simulink model "Digital-Memory-Architecture"  (R2024b)
settings: Solver=VariableStepAuto  StartTime=0.0  StopTime=10.0  RelTol=1e-3
libraries: simulink_extras x129
(part 1 of 5)
settings Model: Creator=suhanoner  LastModifiedBy=suhanoner

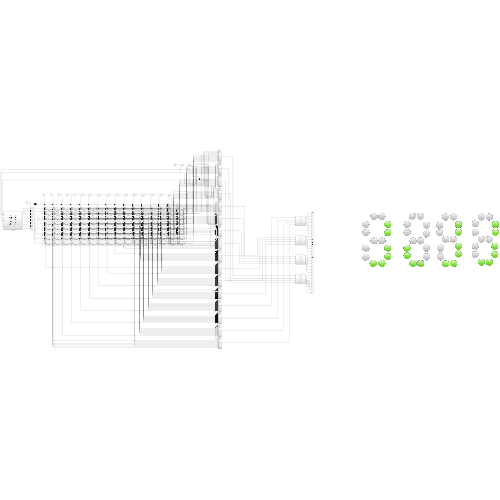
[thumbnail: Simulink's stored preview of the top-level diagram]
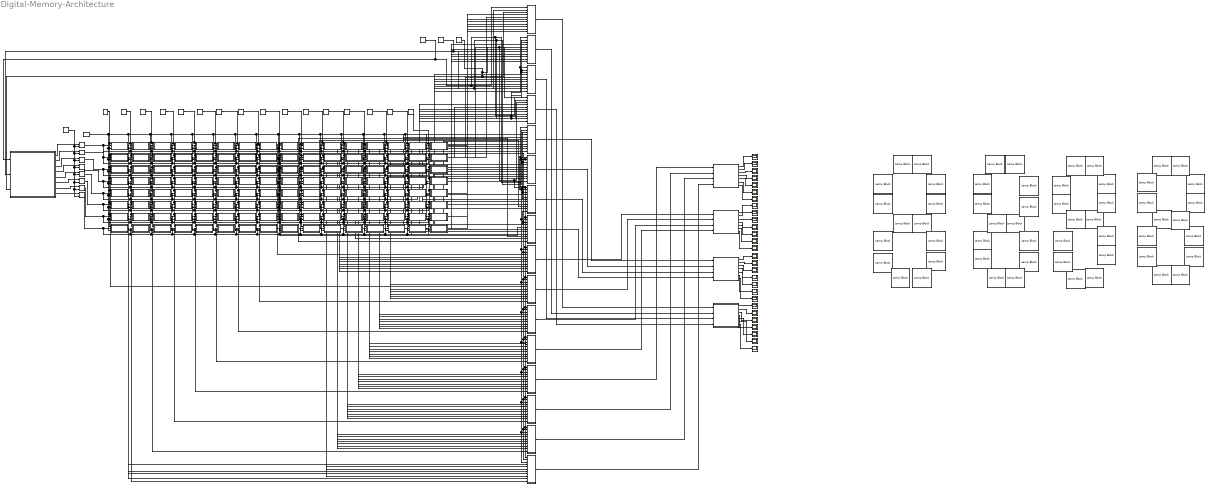
== system Digital-Memory-Architecture ==
  3 to 8 Decoder : Subsystem
  8to1MUX : Subsystem
  8to1MUX1 : Subsystem
  8to1MUX10 : Subsystem
  8to1MUX11 : Subsystem
  8to1MUX12 : Subsystem
  8to1MUX13 : Subsystem
  8to1MUX14 : Subsystem
  8to1MUX15 : Subsystem
  8to1MUX2 : Subsystem
  8to1MUX3 : Subsystem
  8to1MUX4 : Subsystem
  8to1MUX5 : Subsystem
  8to1MUX6 : Subsystem
  8to1MUX7 : Subsystem
  8to1MUX8 : Subsystem
  8to1MUX9 : Subsystem
  Adress0 : Constant
  Adress1 : Constant  Value=0
  Adress2 : Constant  Value=0
  BitCell1 : Subsystem
  BitCell10 : Subsystem
  BitCell100 : Subsystem
  BitCell101 : Subsystem
  BitCell102 : Subsystem
  BitCell103 : Subsystem
  BitCell104 : Subsystem
  BitCell105 : Subsystem
  BitCell106 : Subsystem
  BitCell107 : Subsystem
  BitCell108 : Subsystem
  BitCell109 : Subsystem
  BitCell11 : Subsystem
  BitCell110 : Subsystem
  BitCell111 : Subsystem
  BitCell112 : Subsystem
  BitCell113 : Subsystem
  BitCell114 : Subsystem
  BitCell115 : Subsystem
  BitCell116 : Subsystem
  BitCell117 : Subsystem
  BitCell118 : Subsystem
  BitCell119 : Subsystem
  BitCell12 : Subsystem
  BitCell120 : Subsystem
  BitCell121 : Subsystem
  BitCell122 : Subsystem
  BitCell123 : Subsystem
  BitCell124 : Subsystem
  BitCell125 : Subsystem
  BitCell126 : Subsystem
  BitCell127 : Subsystem
  BitCell128 : Subsystem
  BitCell13 : Subsystem
  BitCell14 : Subsystem
  BitCell15 : Subsystem
  BitCell16 : Subsystem
  BitCell17 : Subsystem
  BitCell18 : Subsystem
  BitCell19 : Subsystem
  BitCell2 : Subsystem
  BitCell20 : Subsystem
  BitCell21 : Subsystem
  BitCell22 : Subsystem
  BitCell23 : Subsystem
  BitCell24 : Subsystem
  BitCell25 : Subsystem
  BitCell26 : Subsystem
  BitCell27 : Subsystem
  BitCell28 : Subsystem
  BitCell29 : Subsystem
  BitCell3 : Subsystem
  BitCell30 : Subsystem
  BitCell31 : Subsystem
  BitCell32 : Subsystem
  BitCell33 : Subsystem
  BitCell34 : Subsystem
  BitCell35 : Subsystem
  BitCell36 : Subsystem
  BitCell37 : Subsystem
  BitCell38 : Subsystem
  BitCell39 : Subsystem
  BitCell4 : Subsystem
  BitCell40 : Subsystem
  BitCell41 : Subsystem
  BitCell42 : Subsystem
  BitCell43 : Subsystem
  BitCell44 : Subsystem
  BitCell45 : Subsystem
  BitCell46 : Subsystem
  BitCell47 : Subsystem
  BitCell48 : Subsystem
  BitCell49 : Subsystem
  BitCell5 : Subsystem
  BitCell50 : Subsystem
  BitCell51 : Subsystem
  BitCell52 : Subsystem
  BitCell53 : Subsystem
  BitCell54 : Subsystem
  BitCell55 : Subsystem
  BitCell56 : Subsystem
  BitCell57 : Subsystem
  BitCell58 : Subsystem
  BitCell59 : Subsystem
  BitCell6 : Subsystem
  BitCell60 : Subsystem
  BitCell61 : Subsystem
  BitCell62 : Subsystem
  BitCell63 : Subsystem
  BitCell64 : Subsystem
  BitCell65 : Subsystem
  BitCell66 : Subsystem
  BitCell67 : Subsystem
  BitCell68 : Subsystem
  BitCell69 : Subsystem
  BitCell7 : Subsystem
  BitCell70 : Subsystem
  BitCell71 : Subsystem
  BitCell72 : Subsystem
  BitCell73 : Subsystem
  BitCell74 : Subsystem
  BitCell75 : Subsystem
  BitCell76 : Subsystem
  BitCell77 : Subsystem
  BitCell78 : Subsystem
  BitCell79 : Subsystem
  BitCell8 : Subsystem
  BitCell80 : Subsystem
  BitCell81 : Subsystem
  BitCell82 : Subsystem
  BitCell83 : Subsystem
  BitCell84 : Subsystem
  BitCell85 : Subsystem
  BitCell86 : Subsystem
  BitCell87 : Subsystem
  BitCell88 : Subsystem
  BitCell89 : Subsystem
  BitCell9 : Subsystem
  BitCell90 : Subsystem
  BitCell91 : Subsystem
  BitCell92 : Subsystem
  BitCell93 : Subsystem
  BitCell94 : Subsystem
  BitCell95 : Subsystem
  BitCell96 : Subsystem
  BitCell97 : Subsystem
  BitCell98 : Subsystem
  BitCell99 : Subsystem
  Clock : simulink_extras/Flip Flops/Clock  period=2
  D_in{,1..4,7..15} (14 alike) : Constant
  D_in5 : Constant  Value=0
  D_in6 : Constant  Value=0
  Lamp{,1..55} (56 alike) : LampBlock  LabelPosition=Hide
  Logical Operator{,1..7} (8 alike) : Logic  AllPortsSameDT=off  OutDataTypeStr=boolean
  R/W : Constant
  Scope{,1..27} (28 alike) : Scope
  Subsystem2 : Subsystem
  Subsystem3 : Subsystem
  Subsystem4 : Subsystem
  Subsystem5 : Subsystem
  wires:
  3 to 8 Decoder/1(Y0) -> Logical Operator/1
  3 to 8 Decoder/2(Y1) -> Logical Operator1/1
  3 to 8 Decoder/3(Y2) -> Logical Operator2/1
  3 to 8 Decoder/4(Y3) -> Logical Operator3/1
  3 to 8 Decoder/5(Y4) -> Logical Operator4/1
  3 to 8 Decoder/6(Y5) -> Logical Operator5/1
  3 to 8 Decoder/7(Y6) -> Logical Operator6/1
  3 to 8 Decoder/8(Y7) -> Logical Operator7/1
  R/W/1 -> Logical Operator7/2, Logical Operator6/2, Logical Operator5/2, Logical Operator4/2, Logical Operator3/2, Logical Operator2/2, Logical Operator1/2, Logical Operator/2
  D_in/1 -> BitCell1/1(D), BitCell9/1(D), BitCell17/1(D), BitCell25/1(D), BitCell33/1(D), BitCell41/1(D), BitCell57/1(D), BitCell49/1(D)
  D_in1/1 -> BitCell2/1(D), BitCell10/1(D), BitCell18/1(D), BitCell26/1(D), BitCell34/1(D), BitCell42/1(D), BitCell58/1(D), BitCell50/1(D)
  D_in2/1 -> BitCell3/1(D), BitCell11/1(D), BitCell19/1(D), BitCell27/1(D), BitCell35/1(D), BitCell43/1(D), BitCell59/1(D), BitCell51/1(D)
  D_in8/1 -> BitCell64/1(D), BitCell100/1(D), BitCell15/1(D), BitCell24/1(D), BitCell39/1(D), BitCell48/1(D), BitCell128/1(D), BitCell91/1(D)
  D_in10/1 -> BitCell102/1(D), BitCell67/1(D), BitCell75/1(D), BitCell83/1(D), BitCell87/1(D), BitCell98/1(D), BitCell110/1(D), BitCell119/1(D)
  Logical Operator/1 -> BitCell1/2(WE), BitCell2/2(WE), BitCell3/2(WE), BitCell4/2(WE), BitCell5/2(WE), BitCell46/2(WE), BitCell55/2(WE), BitCell65/2(WE), BitCell64/2(WE), BitCell93/2(WE), BitCell102/2(WE), BitCell101/2(WE), BitCell99/2(WE), BitCell125/2(WE), BitCell71/2(WE), BitCell70/2(WE)
  Logical Operator4/1 -> BitCell33/2(WE), BitCell34/2(WE), BitCell35/2(WE), BitCell36/2(WE), BitCell37/2(WE), BitCell30/2(WE), BitCell40/2(WE), BitCell47/2(WE), BitCell39/2(WE), BitCell85/2(WE), BitCell87/2(WE), BitCell84/2(WE), BitCell96/2(WE), BitCell120/2(WE), BitCell122/2(WE), BitCell116/2(WE)
  Logical Operator2/1 -> BitCell17/2(WE), BitCell18/2(WE), BitCell19/2(WE), BitCell20/2(WE), BitCell21/2(WE), BitCell14/2(WE), BitCell16/2(WE), BitCell23/2(WE), BitCell15/2(WE), BitCell74/2(WE), BitCell75/2(WE), BitCell68/2(WE), BitCell90/2(WE), BitCell107/2(WE), BitCell109/2(WE), BitCell106/2(WE)
  Logical Operator6/1 -> BitCell49/2(WE), BitCell50/2(WE), BitCell51/2(WE), BitCell52/2(WE), BitCell53/2(WE), BitCell54/2(WE), BitCell73/2(WE), BitCell82/2(WE), BitCell91/2(WE), BitCell103/2(WE), BitCell110/2(WE), BitCell111/2(WE), BitCell123/2(WE), BitCell72/2(WE), BitCell79/2(WE), BitCell78/2(WE)
  Logical Operator7/1 -> BitCell57/2(WE), BitCell58/2(WE), BitCell59/2(WE), BitCell60/2(WE), BitCell61/2(WE), BitCell62/2(WE), BitCell108/2(WE), BitCell117/2(WE), BitCell128/2(WE), BitCell118/2(WE), BitCell119/2(WE), BitCell121/2(WE), BitCell89/2(WE), BitCell81/2(WE), BitCell86/2(WE), BitCell88/2(WE)
  Clock/1 -> BitCell70/3(CLK), BitCell80/3(CLK), BitCell106/3(CLK), BitCell113/3(CLK), BitCell116/3(CLK), BitCell124/3(CLK), BitCell79/3(CLK), BitCell88/3(CLK), BitCell71/3(CLK), BitCell105/3(CLK), BitCell109/3(CLK), BitCell115/3(CLK), BitCell122/3(CLK), BitCell127/3(CLK), BitCell78/3(CLK), BitCell86/3(CLK), BitCell125/3(CLK), BitCell104/3(CLK), BitCell107/3(CLK), BitCell114/3(CLK), BitCell120/3(CLK), BitCell126/3(CLK), BitCell72/3(CLK), BitCell81/3(CLK), BitCell99/3(CLK), BitCell69/3(CLK), BitCell90/3(CLK), BitCell95/3(CLK), BitCell96/3(CLK), BitCell97/3(CLK), BitCell123/3(CLK), BitCell89/3(CLK), BitCell101/3(CLK), BitCell112/3(CLK), BitCell68/3(CLK), BitCell76/3(CLK), BitCell84/3(CLK), BitCell92/3(CLK), BitCell111/3(CLK), BitCell121/3(CLK), BitCell102/3(CLK), BitCell67/3(CLK), BitCell75/3(CLK), BitCell83/3(CLK), BitCell87/3(CLK), BitCell98/3(CLK), BitCell110/3(CLK), BitCell119/3(CLK), BitCell93/3(CLK), BitCell66/3(CLK), BitCell74/3(CLK), BitCell77/3(CLK), BitCell85/3(CLK), BitCell94/3(CLK), BitCell103/3(CLK), BitCell118/3(CLK), BitCell64/3(CLK), BitCell100/3(CLK), BitCell15/3(CLK), BitCell24/3(CLK), BitCell39/3(CLK), BitCell48/3(CLK), BitCell128/3(CLK), BitCell91/3(CLK), BitCell65/3(CLK), BitCell8/3(CLK), BitCell23/3(CLK), BitCell32/3(CLK), BitCell47/3(CLK), BitCell63/3(CLK), BitCell117/3(CLK), BitCell82/3(CLK), BitCell55/3(CLK), BitCell7/3(CLK), BitCell16/3(CLK), BitCell31/3(CLK), BitCell40/3(CLK), BitCell56/3(CLK), BitCell108/3(CLK), BitCell73/3(CLK), BitCell46/3(CLK), BitCell6/3(CLK), BitCell14/3(CLK), BitCell22/3(CLK), BitCell30/3(CLK), BitCell38/3(CLK), BitCell62/3(CLK), BitCell54/3(CLK), BitCell5/3(CLK), BitCell13/3(CLK), BitCell21/3(CLK), BitCell29/3(CLK), BitCell37/3(CLK), BitCell45/3(CLK), BitCell61/3(CLK), BitCell53/3(CLK), BitCell4/3(CLK), BitCell12/3(CLK), BitCell20/3(CLK), BitCell28/3(CLK), BitCell36/3(CLK), BitCell44/3(CLK), BitCell60/3(CLK), BitCell52/3(CLK), BitCell3/3(CLK), BitCell11/3(CLK), BitCell19/3(CLK), BitCell27/3(CLK), BitCell35/3(CLK), BitCell43/3(CLK), BitCell59/3(CLK), BitCell51/3(CLK), BitCell2/3(CLK), BitCell10/3(CLK), BitCell18/3(CLK), BitCell26/3(CLK), BitCell34/3(CLK), BitCell42/3(CLK), BitCell58/3(CLK), BitCell50/3(CLK), BitCell1/3(CLK), BitCell9/3(CLK), BitCell17/3(CLK), BitCell25/3(CLK), BitCell33/3(CLK), BitCell41/3(CLK), BitCell57/3(CLK), BitCell49/3(CLK)
  Logical Operator1/1 -> BitCell9/2(WE), BitCell10/2(WE), BitCell11/2(WE), BitCell12/2(WE), BitCell13/2(WE), BitCell6/2(WE), BitCell7/2(WE), BitCell8/2(WE), BitCell100/2(WE), BitCell66/2(WE), BitCell67/2(WE), BitCell112/2(WE), BitCell69/2(WE), BitCell104/2(WE), BitCell80/2(WE), BitCell105/2(WE)
  Logical Operator3/1 -> BitCell25/2(WE), BitCell26/2(WE), BitCell27/2(WE), BitCell28/2(WE), BitCell29/2(WE), BitCell22/2(WE), BitCell31/2(WE), BitCell32/2(WE), BitCell24/2(WE), BitCell77/2(WE), BitCell83/2(WE), BitCell76/2(WE), BitCell95/2(WE), BitCell114/2(WE), BitCell115/2(WE), BitCell113/2(WE)
  Logical Operator5/1 -> BitCell41/2(WE), BitCell42/2(WE), BitCell43/2(WE), BitCell44/2(WE), BitCell45/2(WE), BitCell38/2(WE), BitCell56/2(WE), BitCell63/2(WE), BitCell48/2(WE), BitCell94/2(WE), BitCell98/2(WE), BitCell92/2(WE), BitCell97/2(WE), BitCell126/2(WE), BitCell127/2(WE), BitCell124/2(WE)
  D_in9/1 -> BitCell93/1(D), BitCell66/1(D), BitCell74/1(D), BitCell77/1(D), BitCell85/1(D), BitCell94/1(D), BitCell103/1(D), BitCell118/1(D)
  D_in3/1 -> BitCell12/1(D), BitCell20/1(D), BitCell28/1(D), BitCell36/1(D), BitCell44/1(D), BitCell60/1(D), BitCell52/1(D), BitCell4/1(D)
  D_in4/1 -> BitCell5/1(D), BitCell13/1(D), BitCell21/1(D), BitCell29/1(D), BitCell37/1(D), BitCell45/1(D), BitCell61/1(D), BitCell53/1(D)
  D_in5/1 -> BitCell6/1(D), BitCell14/1(D), BitCell22/1(D), BitCell30/1(D), BitCell38/1(D), BitCell54/1(D), BitCell62/1(D), BitCell46/1(D)
  D_in6/1 -> BitCell7/1(D), BitCell16/1(D), BitCell31/1(D), BitCell40/1(D), BitCell56/1(D), BitCell108/1(D), BitCell73/1(D), BitCell55/1(D)
  D_in7/1 -> BitCell8/1(D), BitCell23/1(D), BitCell32/1(D), BitCell47/1(D), BitCell63/1(D), BitCell117/1(D), BitCell82/1(D), BitCell65/1(D)
  D_in13/1 -> BitCell125/1(D), BitCell104/1(D), BitCell107/1(D), BitCell114/1(D), BitCell120/1(D), BitCell126/1(D), BitCell72/1(D), BitCell81/1(D)
  D_in14/1 -> BitCell105/1(D), BitCell109/1(D), BitCell115/1(D), BitCell122/1(D), BitCell127/1(D), BitCell86/1(D), BitCell78/1(D), BitCell71/1(D)
  D_in12/1 -> BitCell69/1(D), BitCell90/1(D), BitCell95/1(D), BitCell96/1(D), BitCell97/1(D), BitCell123/1(D), BitCell89/1(D), BitCell99/1(D)
  D_in15/1 -> BitCell80/1(D), BitCell106/1(D), BitCell113/1(D), BitCell116/1(D), BitCell124/1(D), BitCell79/1(D), BitCell88/1(D), BitCell70/1(D)
  D_in11/1 -> BitCell101/1(D), BitCell112/1(D), BitCell68/1(D), BitCell76/1(D), BitCell84/1(D), BitCell92/1(D), BitCell111/1(D), BitCell121/1(D)
  BitCell70/1(Q) -> 8to1MUX/4(D0)
  BitCell80/1(Q) -> 8to1MUX/5(D1)
  BitCell106/1(Q) -> 8to1MUX/6(D2)
  BitCell113/1(Q) -> 8to1MUX/7(D3)
  BitCell116/1(Q) -> 8to1MUX/8(D4)
  BitCell124/1(Q) -> 8to1MUX/9(D5)
  BitCell79/1(Q) -> 8to1MUX/10(D6)
  BitCell88/1(Q) -> 8to1MUX/11(D7)
  BitCell127/1(Q) -> 8to1MUX1/9(D5)
  BitCell122/1(Q) -> 8to1MUX1/8(D4)
  BitCell109/1(Q) -> 8to1MUX1/6(D2)
  BitCell105/1(Q) -> 8to1MUX1/5(D1)
  BitCell115/1(Q) -> 8to1MUX1/7(D3)
  BitCell78/1(Q) -> 8to1MUX1/10(D6)
  BitCell86/1(Q) -> 8to1MUX1/11(D7)
  BitCell71/1(Q) -> 8to1MUX1/4(D0)
  BitCell120/1(Q) -> 8to1MUX2/8(D4)
  BitCell114/1(Q) -> 8to1MUX2/7(D3)
  BitCell107/1(Q) -> 8to1MUX2/6(D2)
  BitCell81/1(Q) -> 8to1MUX2/11(D7)
  BitCell125/1(Q) -> 8to1MUX2/4(D0)
  BitCell104/1(Q) -> 8to1MUX2/5(D1)
  BitCell72/1(Q) -> 8to1MUX2/10(D6)
  BitCell126/1(Q) -> 8to1MUX2/9(D5)
  BitCell96/1(Q) -> 8to1MUX3/8(D4)
  BitCell95/1(Q) -> 8to1MUX3/7(D3)
  BitCell90/1(Q) -> 8to1MUX3/6(D2)
  BitCell89/1(Q) -> 8to1MUX3/11(D7)
  BitCell99/1(Q) -> 8to1MUX3/4(D0)
  BitCell69/1(Q) -> 8to1MUX3/5(D1)
  BitCell123/1(Q) -> 8to1MUX3/10(D6)
  BitCell97/1(Q) -> 8to1MUX3/9(D5)
  BitCell84/1(Q) -> 8to1MUX4/8(D4)
  BitCell76/1(Q) -> 8to1MUX4/7(D3)
  BitCell68/1(Q) -> 8to1MUX4/6(D2)
  BitCell121/1(Q) -> 8to1MUX4/11(D7)
  BitCell101/1(Q) -> 8to1MUX4/4(D0)
  BitCell112/1(Q) -> 8to1MUX4/5(D1)
  BitCell111/1(Q) -> 8to1MUX4/10(D6)
  BitCell92/1(Q) -> 8to1MUX4/9(D5)
  BitCell87/1(Q) -> 8to1MUX5/8(D4)
  BitCell83/1(Q) -> 8to1MUX5/7(D3)
  BitCell75/1(Q) -> 8to1MUX5/6(D2)
  BitCell119/1(Q) -> 8to1MUX5/11(D7)
  BitCell102/1(Q) -> 8to1MUX5/4(D0)
  BitCell67/1(Q) -> 8to1MUX5/5(D1)
  BitCell110/1(Q) -> 8to1MUX5/10(D6)
  BitCell98/1(Q) -> 8to1MUX5/9(D5)
  BitCell85/1(Q) -> 8to1MUX6/8(D4)
  BitCell77/1(Q) -> 8to1MUX6/7(D3)
  BitCell74/1(Q) -> 8to1MUX6/6(D2)
  BitCell118/1(Q) -> 8to1MUX6/11(D7)
  BitCell93/1(Q) -> 8to1MUX6/4(D0)
  BitCell66/1(Q) -> 8to1MUX6/5(D1)
  BitCell103/1(Q) -> 8to1MUX6/10(D6)
  BitCell94/1(Q) -> 8to1MUX6/9(D5)
  Adress1/1 -> 8to1MUX15/3(Adress2), 8to1MUX14/3(Adress2), 8to1MUX13/3(Adress2), 8to1MUX12/3(Adress2), 8to1MUX11/3(Adress2), 8to1MUX10/3(Adress2), 8to1MUX9/3(Adress2), 8to1MUX8/2(Adress1), 8to1MUX7/2(Adress1), 8to1MUX6/2(Adress1), 8to1MUX5/2(Adress1), 8to1MUX4/2(Adress1), 8to1MUX3/2(Adress1), 8to1MUX1/2(Adress1), 8to1MUX2/2(Adress1), 8to1MUX/2(Adress1), 3 to 8 Decoder/2(A1)
  BitCell39/1(Q) -> 8to1MUX7/8(D4)
  BitCell24/1(Q) -> 8to1MUX7/7(D3)
  BitCell15/1(Q) -> 8to1MUX7/6(D2)
  BitCell128/1(Q) -> 8to1MUX7/11(D7)
  BitCell64/1(Q) -> 8to1MUX7/4(D0)
  BitCell100/1(Q) -> 8to1MUX7/5(D1)
  BitCell91/1(Q) -> 8to1MUX7/10(D6)
  Adress2/1 -> 8to1MUX/3(Adress2), 3 to 8 Decoder/3(A2), 8to1MUX2/3(Adress2), 8to1MUX1/3(Adress2), 8to1MUX5/3(Adress2), 8to1MUX4/3(Adress2), 8to1MUX15/2(Adress1), 8to1MUX14/2(Adress1), 8to1MUX13/2(Adress1), 8to1MUX12/2(Adress1), 8to1MUX11/2(Adress1), 8to1MUX10/2(Adress1), 8to1MUX9/2(Adress1), 8to1MUX8/3(Adress2), 8to1MUX7/3(Adress2), 8to1MUX6/3(Adress2), 8to1MUX3/3(Adress2)
  Adress0/1 -> 8to1MUX5/1(Adress0), 8to1MUX4/1(Adress0), 8to1MUX15/1(Adress0), 8to1MUX14/1(Adress0), 8to1MUX13/1(Adress0), 8to1MUX12/1(Adress0), 8to1MUX11/1(Adress0), 8to1MUX10/1(Adress0), 8to1MUX9/1(Adress0), 8to1MUX8/1(Adress0), 8to1MUX7/1(Adress0), 8to1MUX6/1(Adress0), 8to1MUX3/1(Adress0), 8to1MUX1/1(Adress0), 8to1MUX2/1(Adress0), 8to1MUX/1(Adress0), 3 to 8 Decoder/1(A0)
  BitCell48/1(Q) -> 8to1MUX7/9(D5)
  BitCell65/1(Q) -> 8to1MUX8/4(D0)
  BitCell8/1(Q) -> 8to1MUX8/5(D1)
  BitCell23/1(Q) -> 8to1MUX8/6(D2)
  BitCell32/1(Q) -> 8to1MUX8/7(D3)
  BitCell47/1(Q) -> 8to1MUX8/8(D4)
  BitCell63/1(Q) -> 8to1MUX8/9(D5)
  BitCell82/1(Q) -> 8to1MUX8/10(D6)
  BitCell117/1(Q) -> 8to1MUX8/11(D7)
  BitCell55/1(Q) -> 8to1MUX9/4(D0)
  BitCell16/1(Q) -> 8to1MUX9/6(D2)
  BitCell31/1(Q) -> 8to1MUX9/7(D3)
  BitCell40/1(Q) -> 8to1MUX9/8(D4)
  BitCell56/1(Q) -> 8to1MUX9/9(D5)
  BitCell73/1(Q) -> 8to1MUX9/10(D6)
  BitCell108/1(Q) -> 8to1MUX9/11(D7)
  BitCell46/1(Q) -> 8to1MUX10/4(D0)
  BitCell6/1(Q) -> 8to1MUX10/5(D1)
  BitCell14/1(Q) -> 8to1MUX10/6(D2)
  BitCell22/1(Q) -> 8to1MUX10/7(D3)
  BitCell30/1(Q) -> 8to1MUX10/8(D4)
  BitCell38/1(Q) -> 8to1MUX10/9(D5)
  BitCell54/1(Q) -> 8to1MUX10/10(D6)
  BitCell62/1(Q) -> 8to1MUX10/11(D7)
  BitCell5/1(Q) -> 8to1MUX11/4(D0)
  BitCell13/1(Q) -> 8to1MUX11/5(D1)
  BitCell21/1(Q) -> 8to1MUX11/6(D2)
  BitCell29/1(Q) -> 8to1MUX11/7(D3)
  BitCell37/1(Q) -> 8to1MUX11/8(D4)
  BitCell45/1(Q) -> 8to1MUX11/9(D5)
  BitCell53/1(Q) -> 8to1MUX11/10(D6)
  BitCell61/1(Q) -> 8to1MUX11/11(D7)
  BitCell4/1(Q) -> 8to1MUX12/4(D0)
  BitCell12/1(Q) -> 8to1MUX12/5(D1)
  BitCell20/1(Q) -> 8to1MUX12/6(D2)
  BitCell28/1(Q) -> 8to1MUX12/7(D3)
  BitCell36/1(Q) -> 8to1MUX12/8(D4)
  BitCell44/1(Q) -> 8to1MUX12/9(D5)
  BitCell52/1(Q) -> 8to1MUX12/10(D6)
  BitCell60/1(Q) -> 8to1MUX12/11(D7)
  BitCell7/1(Q) -> 8to1MUX9/5(D1)
  BitCell3/1(Q) -> 8to1MUX13/4(D0)
  BitCell11/1(Q) -> 8to1MUX13/5(D1)
  BitCell19/1(Q) -> 8to1MUX13/6(D2)
  BitCell27/1(Q) -> 8to1MUX13/7(D3)
  BitCell35/1(Q) -> 8to1MUX13/8(D4)
  BitCell43/1(Q) -> 8to1MUX13/9(D5)
  BitCell51/1(Q) -> 8to1MUX13/10(D6)
  BitCell59/1(Q) -> 8to1MUX13/11(D7)
  BitCell2/1(Q) -> 8to1MUX14/4(D0)
  BitCell10/1(Q) -> 8to1MUX14/5(D1)
  BitCell18/1(Q) -> 8to1MUX14/6(D2)
  BitCell26/1(Q) -> 8to1MUX14/7(D3)
  BitCell34/1(Q) -> 8to1MUX14/8(D4)
  BitCell42/1(Q) -> 8to1MUX14/9(D5)
  BitCell50/1(Q) -> 8to1MUX14/10(D6)
  BitCell58/1(Q) -> 8to1MUX14/11(D7)
  BitCell1/1(Q) -> 8to1MUX15/4(D0)
  BitCell9/1(Q) -> 8to1MUX15/5(D1)
  BitCell17/1(Q) -> 8to1MUX15/6(D2)
  BitCell25/1(Q) -> 8to1MUX15/7(D3)
  BitCell33/1(Q) -> 8to1MUX15/8(D4)
  BitCell41/1(Q) -> 8to1MUX15/9(D5)
  BitCell49/1(Q) -> 8to1MUX15/10(D6)
  BitCell57/1(Q) -> 8to1MUX15/11(D7)
  8to1MUX/1(A) -> Subsystem5/1(A)
  8to1MUX1/1(B) -> Subsystem5/2(B)
  8to1MUX2/1(C) -> Subsystem5/3(C)
  8to1MUX3/1(D) -> Subsystem5/4(D)
  8to1MUX4/1(A) -> Subsystem3/1(A)
  8to1MUX5/1(B) -> Subsystem3/2(B)
  8to1MUX6/1(C) -> Subsystem3/3(C)
  8to1MUX7/1(D) -> Subsystem3/4(D)
  8to1MUX8/1(A) -> Subsystem2/1(A)
  8to1MUX9/1(B) -> Subsystem2/2(B)
  8to1MUX10/1(C) -> Subsystem2/3(C)
  8to1MUX11/1(D) -> Subsystem2/4(D)
  8to1MUX12/1(A) -> Subsystem4/1(A)
  8to1MUX13/1(B) -> Subsystem4/2(B)
  8to1MUX14/1(C) -> Subsystem4/3(C)
  8to1MUX15/1(D) -> Subsystem4/4(D)
  Subsystem4/1(a) -> Scope/1
  Subsystem4/2(b) -> Scope1/1
  Subsystem4/3(c) -> Scope2/1
  Subsystem4/4(d) -> Scope3/1
  Subsystem4/5(e) -> Scope4/1
  Subsystem4/6(f) -> Scope5/1
  Subsystem4/7(g) -> Scope6/1
  Subsystem2/2(b) -> Scope8/1
  Subsystem2/5(e) -> Scope11/1
  Subsystem2/6(f) -> Scope12/1
  Subsystem2/3(c) -> Scope9/1
  Subsystem2/7(g) -> Scope13/1
  Subsystem2/4(d) -> Scope10/1
  Subsystem2/1(a) -> Scope7/1
  Subsystem3/2(b) -> Scope15/1
  Subsystem3/5(e) -> Scope18/1
  Subsystem3/6(f) -> Scope19/1
  Subsystem3/3(c) -> Scope16/1
  Subsystem3/7(g) -> Scope20/1
  Subsystem3/4(d) -> Scope17/1
  Subsystem3/1(a) -> Scope14/1
  Subsystem5/7(g) -> Scope27/1
  Subsystem5/6(f) -> Scope26/1
  Subsystem5/5(e) -> Scope25/1
  Subsystem5/4(d) -> Scope24/1
  Subsystem5/3(c) -> Scope23/1
  Subsystem5/2(b) -> Scope22/1
  Subsystem5/1(a) -> Scope21/1

== system Digital-Memory-Architecture/3 to 8 Decoder ==
  A0 : Inport
  A1 : Inport  Port=2
  A2 : Inport  Port=3
  A0' : Logic  Operator=NOT  AllPortsSameDT=off  OutDataTypeStr=boolean
  A1' : Logic  Operator=NOT  AllPortsSameDT=off  OutDataTypeStr=boolean
  A2' : Logic  Operator=NOT  AllPortsSameDT=off  OutDataTypeStr=boolean
  Logical Operator{,1..7} (8 alike) : Logic  Inputs=3  AllPortsSameDT=off  OutDataTypeStr=boolean
  Y0 : Outport
  Y1 : Outport  Port=2
  Y2 : Outport  Port=3
  Y3 : Outport  Port=4
  Y4 : Outport  Port=5
  Y5 : Outport  Port=6
  Y6 : Outport  Port=7
  Y7 : Outport  Port=8
  wires:
  Logical Operator/1 -> Y0/1
  Logical Operator7/1 -> Y7/1
  Logical Operator1/1 -> Y1/1
  A2/1 -> Logical Operator7/3, Logical Operator6/3, Logical Operator5/3, Logical Operator4/3, A2'/1
  Logical Operator5/1 -> Y5/1
  A0'/1 -> Logical Operator6/1, Logical Operator4/1, Logical Operator2/1, Logical Operator/1
  A1/1 -> Logical Operator2/2, Logical Operator3/2, A1'/1, Logical Operator6/2, Logical Operator7/2
  Logical Operator4/1 -> Y4/1
  Logical Operator2/1 -> Y2/1
  A0/1 -> Logical Operator7/1, Logical Operator5/1, Logical Operator3/1, Logical Operator1/1, A0'/1
  Logical Operator3/1 -> Y3/1
  A1'/1 -> Logical Operator4/2, Logical Operator5/2, Logical Operator1/2, Logical Operator/2
  A2'/1 -> Logical Operator3/3, Logical Operator2/3, Logical Operator1/3, Logical Operator/3
  Logical Operator6/1 -> Y6/1

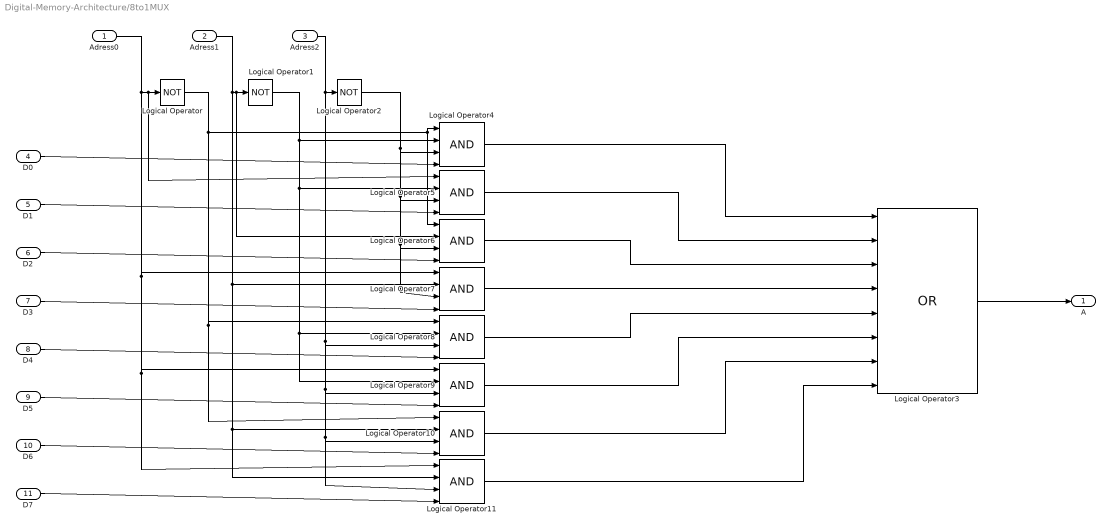
== system Digital-Memory-Architecture/8to1MUX ==
  Adress0 : Inport
  Adress1 : Inport  Port=2
  Adress2 : Inport  Port=3
  D0 : Inport  Port=4
  D1 : Inport  Port=5
  D2 : Inport  Port=6
  D3 : Inport  Port=7
  D4 : Inport  Port=8
  D5 : Inport  Port=9
  D6 : Inport  Port=10
  D7 : Inport  Port=11
  Logical Operator : Logic  Operator=NOT  IconShape=distinctive  AllPortsSameDT=off  OutDataTypeStr=boolean
  Logical Operator1 : Logic  Operator=NOT  IconShape=distinctive  AllPortsSameDT=off  OutDataTypeStr=boolean
  Logical Operator{4..11} (8 alike) : Logic  Inputs=4  IconShape=distinctive  AllPortsSameDT=off  OutDataTypeStr=boolean
  Logical Operator2 : Logic  Operator=NOT  IconShape=distinctive  AllPortsSameDT=off  OutDataTypeStr=boolean
  Logical Operator3 : Logic  Operator=OR  Inputs=8  IconShape=distinctive  AllPortsSameDT=off  OutDataTypeStr=boolean
  A : Outport
  wires:
  Logical Operator3/1 -> A/1
  Adress0/1 -> Logical Operator11/1, Logical Operator9/1, Logical Operator7/1, Logical Operator5/1, Logical Operator/1
  Adress1/1 -> Logical Operator11/2, Logical Operator10/2, Logical Operator7/2, Logical Operator6/2, Logical Operator1/1
  Adress2/1 -> Logical Operator11/3, Logical Operator10/3, Logical Operator9/3, Logical Operator8/3, Logical Operator2/1
  D7/1 -> Logical Operator11/4
  D6/1 -> Logical Operator10/4
  D5/1 -> Logical Operator9/4
  D4/1 -> Logical Operator8/4
  D3/1 -> Logical Operator7/4
  D2/1 -> Logical Operator6/4
  D1/1 -> Logical Operator5/4
  D0/1 -> Logical Operator4/4
  Logical Operator2/1 -> Logical Operator7/3, Logical Operator6/3, Logical Operator5/3, Logical Operator4/3
  Logical Operator1/1 -> Logical Operator9/2, Logical Operator8/2, Logical Operator5/2, Logical Operator4/2
  Logical Operator/1 -> Logical Operator10/1, Logical Operator8/1, Logical Operator6/1, Logical Operator4/1
  Logical Operator4/1 -> Logical Operator3/1
  Logical Operator5/1 -> Logical Operator3/2
  Logical Operator6/1 -> Logical Operator3/3
  Logical Operator7/1 -> Logical Operator3/4
  Logical Operator8/1 -> Logical Operator3/5
  Logical Operator9/1 -> Logical Operator3/6
  Logical Operator10/1 -> Logical Operator3/7
  Logical Operator11/1 -> Logical Operator3/8

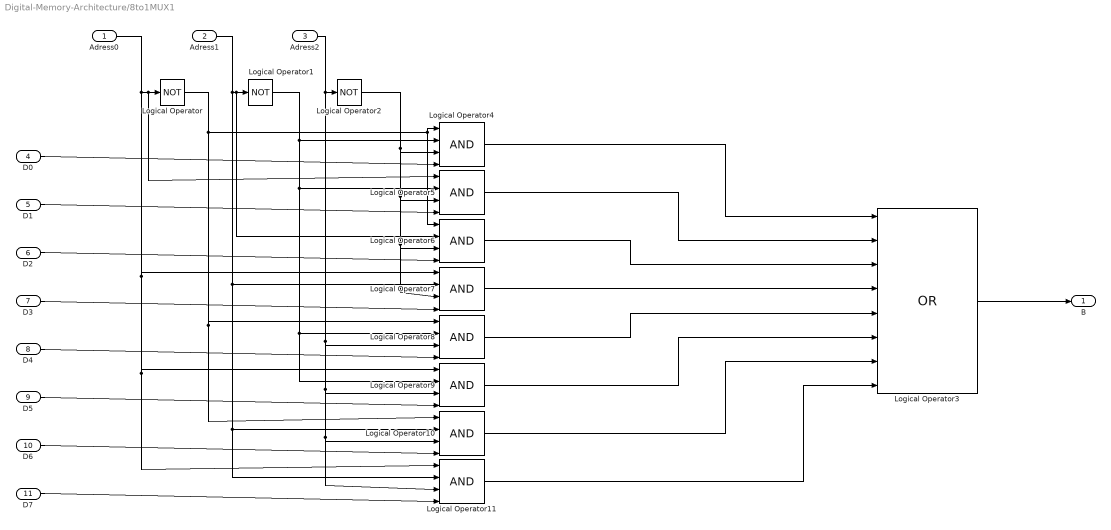
== system Digital-Memory-Architecture/8to1MUX1 ==
  Adress0 : Inport
  Adress1 : Inport  Port=2
  Adress2 : Inport  Port=3
  D0 : Inport  Port=4
  D1 : Inport  Port=5
  D2 : Inport  Port=6
  D3 : Inport  Port=7
  D4 : Inport  Port=8
  D5 : Inport  Port=9
  D6 : Inport  Port=10
  D7 : Inport  Port=11
  Logical Operator : Logic  Operator=NOT  IconShape=distinctive  AllPortsSameDT=off  OutDataTypeStr=boolean
  Logical Operator1 : Logic  Operator=NOT  IconShape=distinctive  AllPortsSameDT=off  OutDataTypeStr=boolean
  Logical Operator{4..11} (8 alike) : Logic  Inputs=4  IconShape=distinctive  AllPortsSameDT=off  OutDataTypeStr=boolean
  Logical Operator2 : Logic  Operator=NOT  IconShape=distinctive  AllPortsSameDT=off  OutDataTypeStr=boolean
  Logical Operator3 : Logic  Operator=OR  Inputs=8  IconShape=distinctive  AllPortsSameDT=off  OutDataTypeStr=boolean
  B : Outport
  wires:
  Logical Operator3/1 -> B/1
  Adress0/1 -> Logical Operator11/1, Logical Operator9/1, Logical Operator7/1, Logical Operator5/1, Logical Operator/1
  Adress1/1 -> Logical Operator11/2, Logical Operator10/2, Logical Operator7/2, Logical Operator6/2, Logical Operator1/1
  Adress2/1 -> Logical Operator11/3, Logical Operator10/3, Logical Operator9/3, Logical Operator8/3, Logical Operator2/1
  D7/1 -> Logical Operator11/4
  D6/1 -> Logical Operator10/4
  D5/1 -> Logical Operator9/4
  D4/1 -> Logical Operator8/4
  D3/1 -> Logical Operator7/4
  D2/1 -> Logical Operator6/4
  D1/1 -> Logical Operator5/4
  D0/1 -> Logical Operator4/4
  Logical Operator2/1 -> Logical Operator7/3, Logical Operator6/3, Logical Operator5/3, Logical Operator4/3
  Logical Operator1/1 -> Logical Operator9/2, Logical Operator8/2, Logical Operator5/2, Logical Operator4/2
  Logical Operator/1 -> Logical Operator10/1, Logical Operator8/1, Logical Operator6/1, Logical Operator4/1
  Logical Operator4/1 -> Logical Operator3/1
  Logical Operator5/1 -> Logical Operator3/2
  Logical Operator6/1 -> Logical Operator3/3
  Logical Operator7/1 -> Logical Operator3/4
  Logical Operator8/1 -> Logical Operator3/5
  Logical Operator9/1 -> Logical Operator3/6
  Logical Operator10/1 -> Logical Operator3/7
  Logical Operator11/1 -> Logical Operator3/8

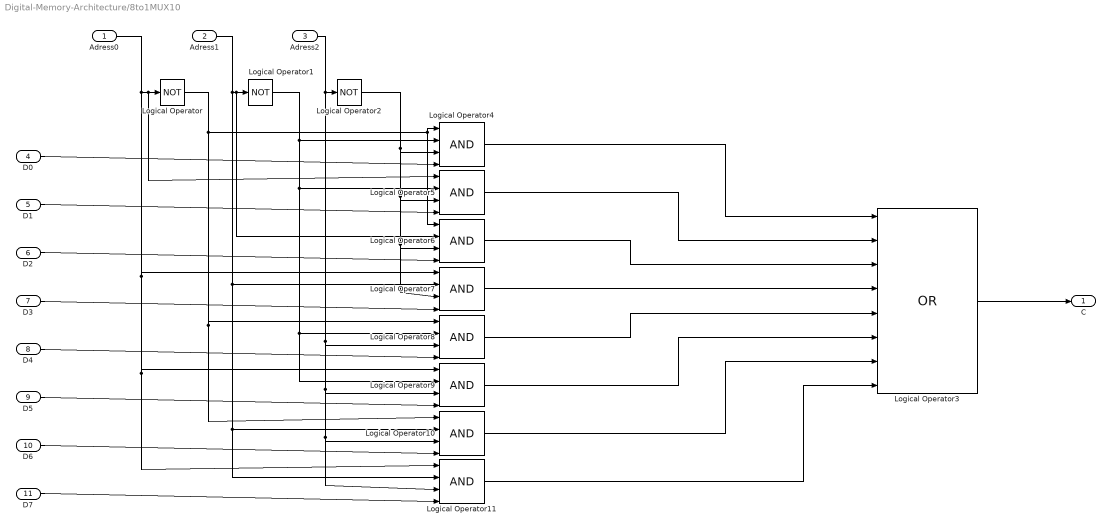
== system Digital-Memory-Architecture/8to1MUX10 ==
  Adress0 : Inport
  Adress1 : Inport  Port=2
  Adress2 : Inport  Port=3
  D0 : Inport  Port=4
  D1 : Inport  Port=5
  D2 : Inport  Port=6
  D3 : Inport  Port=7
  D4 : Inport  Port=8
  D5 : Inport  Port=9
  D6 : Inport  Port=10
  D7 : Inport  Port=11
  Logical Operator : Logic  Operator=NOT  IconShape=distinctive  AllPortsSameDT=off  OutDataTypeStr=boolean
  Logical Operator1 : Logic  Operator=NOT  IconShape=distinctive  AllPortsSameDT=off  OutDataTypeStr=boolean
  Logical Operator{4..11} (8 alike) : Logic  Inputs=4  IconShape=distinctive  AllPortsSameDT=off  OutDataTypeStr=boolean
  Logical Operator2 : Logic  Operator=NOT  IconShape=distinctive  AllPortsSameDT=off  OutDataTypeStr=boolean
  Logical Operator3 : Logic  Operator=OR  Inputs=8  IconShape=distinctive  AllPortsSameDT=off  OutDataTypeStr=boolean
  C : Outport
  wires:
  Logical Operator3/1 -> C/1
  Adress0/1 -> Logical Operator11/1, Logical Operator9/1, Logical Operator7/1, Logical Operator5/1, Logical Operator/1
  Adress1/1 -> Logical Operator11/2, Logical Operator10/2, Logical Operator7/2, Logical Operator6/2, Logical Operator1/1
  Adress2/1 -> Logical Operator11/3, Logical Operator10/3, Logical Operator9/3, Logical Operator8/3, Logical Operator2/1
  D7/1 -> Logical Operator11/4
  D6/1 -> Logical Operator10/4
  D5/1 -> Logical Operator9/4
  D4/1 -> Logical Operator8/4
  D3/1 -> Logical Operator7/4
  D2/1 -> Logical Operator6/4
  D1/1 -> Logical Operator5/4
  D0/1 -> Logical Operator4/4
  Logical Operator2/1 -> Logical Operator7/3, Logical Operator6/3, Logical Operator5/3, Logical Operator4/3
  Logical Operator1/1 -> Logical Operator9/2, Logical Operator8/2, Logical Operator5/2, Logical Operator4/2
  Logical Operator/1 -> Logical Operator10/1, Logical Operator8/1, Logical Operator6/1, Logical Operator4/1
  Logical Operator4/1 -> Logical Operator3/1
  Logical Operator5/1 -> Logical Operator3/2
  Logical Operator6/1 -> Logical Operator3/3
  Logical Operator7/1 -> Logical Operator3/4
  Logical Operator8/1 -> Logical Operator3/5
  Logical Operator9/1 -> Logical Operator3/6
  Logical Operator10/1 -> Logical Operator3/7
  Logical Operator11/1 -> Logical Operator3/8

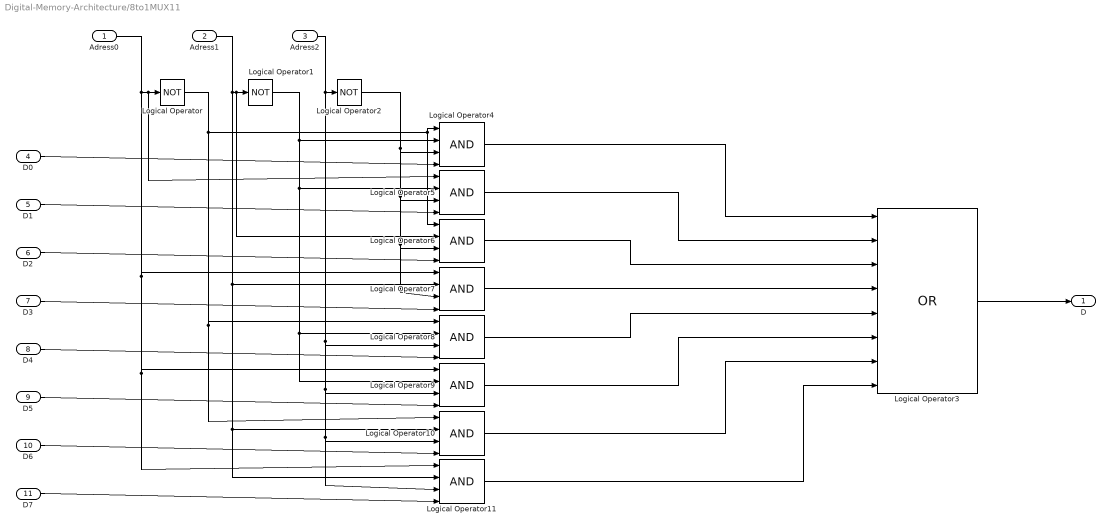
== system Digital-Memory-Architecture/8to1MUX11 ==
  Adress0 : Inport
  Adress1 : Inport  Port=2
  Adress2 : Inport  Port=3
  D0 : Inport  Port=4
  D1 : Inport  Port=5
  D2 : Inport  Port=6
  D3 : Inport  Port=7
  D4 : Inport  Port=8
  D5 : Inport  Port=9
  D6 : Inport  Port=10
  D7 : Inport  Port=11
  Logical Operator : Logic  Operator=NOT  IconShape=distinctive  AllPortsSameDT=off  OutDataTypeStr=boolean
  Logical Operator1 : Logic  Operator=NOT  IconShape=distinctive  AllPortsSameDT=off  OutDataTypeStr=boolean
  Logical Operator{4..11} (8 alike) : Logic  Inputs=4  IconShape=distinctive  AllPortsSameDT=off  OutDataTypeStr=boolean
  Logical Operator2 : Logic  Operator=NOT  IconShape=distinctive  AllPortsSameDT=off  OutDataTypeStr=boolean
  Logical Operator3 : Logic  Operator=OR  Inputs=8  IconShape=distinctive  AllPortsSameDT=off  OutDataTypeStr=boolean
  D : Outport
  wires:
  Logical Operator3/1 -> D/1
  Adress0/1 -> Logical Operator11/1, Logical Operator9/1, Logical Operator7/1, Logical Operator5/1, Logical Operator/1
  Adress1/1 -> Logical Operator11/2, Logical Operator10/2, Logical Operator7/2, Logical Operator6/2, Logical Operator1/1
  Adress2/1 -> Logical Operator11/3, Logical Operator10/3, Logical Operator9/3, Logical Operator8/3, Logical Operator2/1
  D7/1 -> Logical Operator11/4
  D6/1 -> Logical Operator10/4
  D5/1 -> Logical Operator9/4
  D4/1 -> Logical Operator8/4
  D3/1 -> Logical Operator7/4
  D2/1 -> Logical Operator6/4
  D1/1 -> Logical Operator5/4
  D0/1 -> Logical Operator4/4
  Logical Operator2/1 -> Logical Operator7/3, Logical Operator6/3, Logical Operator5/3, Logical Operator4/3
  Logical Operator1/1 -> Logical Operator9/2, Logical Operator8/2, Logical Operator5/2, Logical Operator4/2
  Logical Operator/1 -> Logical Operator10/1, Logical Operator8/1, Logical Operator6/1, Logical Operator4/1
  Logical Operator4/1 -> Logical Operator3/1
  Logical Operator5/1 -> Logical Operator3/2
  Logical Operator6/1 -> Logical Operator3/3
  Logical Operator7/1 -> Logical Operator3/4
  Logical Operator8/1 -> Logical Operator3/5
  Logical Operator9/1 -> Logical Operator3/6
  Logical Operator10/1 -> Logical Operator3/7
  Logical Operator11/1 -> Logical Operator3/8

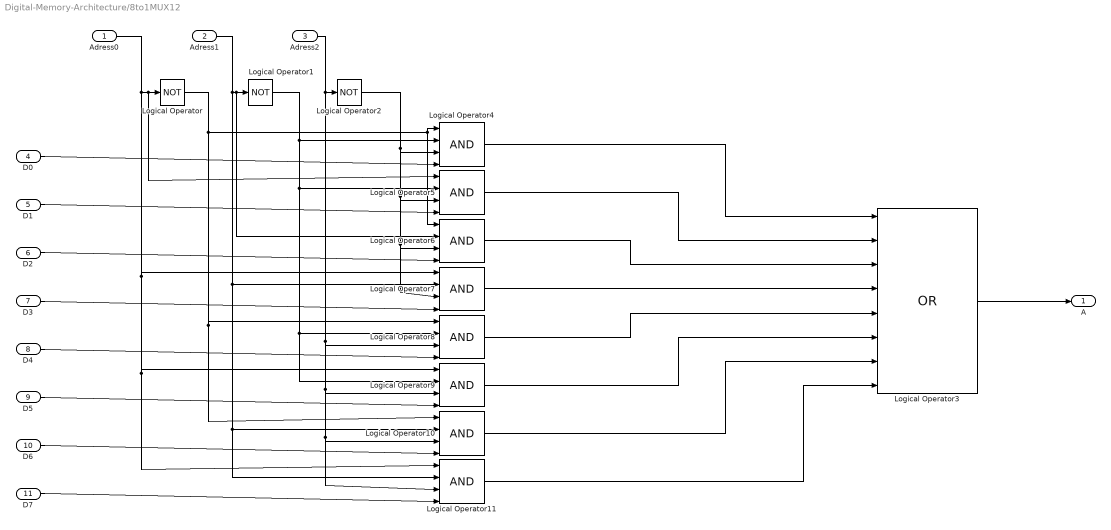
== system Digital-Memory-Architecture/8to1MUX12 ==
  Adress0 : Inport
  Adress1 : Inport  Port=2
  Adress2 : Inport  Port=3
  D0 : Inport  Port=4
  D1 : Inport  Port=5
  D2 : Inport  Port=6
  D3 : Inport  Port=7
  D4 : Inport  Port=8
  D5 : Inport  Port=9
  D6 : Inport  Port=10
  D7 : Inport  Port=11
  Logical Operator : Logic  Operator=NOT  IconShape=distinctive  AllPortsSameDT=off  OutDataTypeStr=boolean
  Logical Operator1 : Logic  Operator=NOT  IconShape=distinctive  AllPortsSameDT=off  OutDataTypeStr=boolean
  Logical Operator{4..11} (8 alike) : Logic  Inputs=4  IconShape=distinctive  AllPortsSameDT=off  OutDataTypeStr=boolean
  Logical Operator2 : Logic  Operator=NOT  IconShape=distinctive  AllPortsSameDT=off  OutDataTypeStr=boolean
  Logical Operator3 : Logic  Operator=OR  Inputs=8  IconShape=distinctive  AllPortsSameDT=off  OutDataTypeStr=boolean
  A : Outport
  wires:
  Logical Operator3/1 -> A/1
  Adress0/1 -> Logical Operator11/1, Logical Operator9/1, Logical Operator7/1, Logical Operator5/1, Logical Operator/1
  Adress1/1 -> Logical Operator11/2, Logical Operator10/2, Logical Operator7/2, Logical Operator6/2, Logical Operator1/1
  Adress2/1 -> Logical Operator11/3, Logical Operator10/3, Logical Operator9/3, Logical Operator8/3, Logical Operator2/1
  D7/1 -> Logical Operator11/4
  D6/1 -> Logical Operator10/4
  D5/1 -> Logical Operator9/4
  D4/1 -> Logical Operator8/4
  D3/1 -> Logical Operator7/4
  D2/1 -> Logical Operator6/4
  D1/1 -> Logical Operator5/4
  D0/1 -> Logical Operator4/4
  Logical Operator2/1 -> Logical Operator7/3, Logical Operator6/3, Logical Operator5/3, Logical Operator4/3
  Logical Operator1/1 -> Logical Operator9/2, Logical Operator8/2, Logical Operator5/2, Logical Operator4/2
  Logical Operator/1 -> Logical Operator10/1, Logical Operator8/1, Logical Operator6/1, Logical Operator4/1
  Logical Operator4/1 -> Logical Operator3/1
  Logical Operator5/1 -> Logical Operator3/2
  Logical Operator6/1 -> Logical Operator3/3
  Logical Operator7/1 -> Logical Operator3/4
  Logical Operator8/1 -> Logical Operator3/5
  Logical Operator9/1 -> Logical Operator3/6
  Logical Operator10/1 -> Logical Operator3/7
  Logical Operator11/1 -> Logical Operator3/8

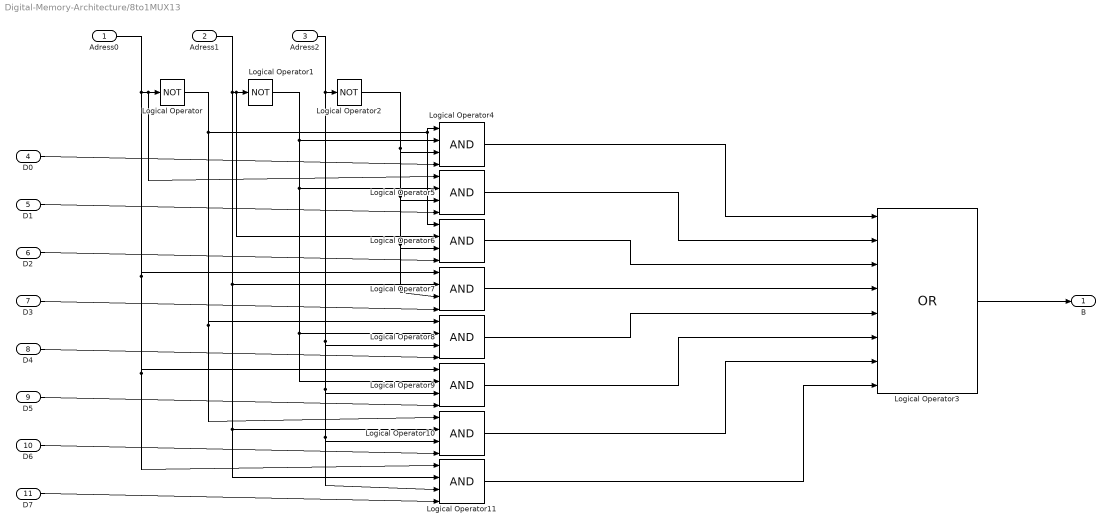
== system Digital-Memory-Architecture/8to1MUX13 ==
  Adress0 : Inport
  Adress1 : Inport  Port=2
  Adress2 : Inport  Port=3
  D0 : Inport  Port=4
  D1 : Inport  Port=5
  D2 : Inport  Port=6
  D3 : Inport  Port=7
  D4 : Inport  Port=8
  D5 : Inport  Port=9
  D6 : Inport  Port=10
  D7 : Inport  Port=11
  Logical Operator : Logic  Operator=NOT  IconShape=distinctive  AllPortsSameDT=off  OutDataTypeStr=boolean
  Logical Operator1 : Logic  Operator=NOT  IconShape=distinctive  AllPortsSameDT=off  OutDataTypeStr=boolean
  Logical Operator{4..11} (8 alike) : Logic  Inputs=4  IconShape=distinctive  AllPortsSameDT=off  OutDataTypeStr=boolean
  Logical Operator2 : Logic  Operator=NOT  IconShape=distinctive  AllPortsSameDT=off  OutDataTypeStr=boolean
  Logical Operator3 : Logic  Operator=OR  Inputs=8  IconShape=distinctive  AllPortsSameDT=off  OutDataTypeStr=boolean
  B : Outport
  wires:
  Logical Operator3/1 -> B/1
  Adress0/1 -> Logical Operator11/1, Logical Operator9/1, Logical Operator7/1, Logical Operator5/1, Logical Operator/1
  Adress1/1 -> Logical Operator11/2, Logical Operator10/2, Logical Operator7/2, Logical Operator6/2, Logical Operator1/1
  Adress2/1 -> Logical Operator11/3, Logical Operator10/3, Logical Operator9/3, Logical Operator8/3, Logical Operator2/1
  D7/1 -> Logical Operator11/4
  D6/1 -> Logical Operator10/4
  D5/1 -> Logical Operator9/4
  D4/1 -> Logical Operator8/4
  D3/1 -> Logical Operator7/4
  D2/1 -> Logical Operator6/4
  D1/1 -> Logical Operator5/4
  D0/1 -> Logical Operator4/4
  Logical Operator2/1 -> Logical Operator7/3, Logical Operator6/3, Logical Operator5/3, Logical Operator4/3
  Logical Operator1/1 -> Logical Operator9/2, Logical Operator8/2, Logical Operator5/2, Logical Operator4/2
  Logical Operator/1 -> Logical Operator10/1, Logical Operator8/1, Logical Operator6/1, Logical Operator4/1
  Logical Operator4/1 -> Logical Operator3/1
  Logical Operator5/1 -> Logical Operator3/2
  Logical Operator6/1 -> Logical Operator3/3
  Logical Operator7/1 -> Logical Operator3/4
  Logical Operator8/1 -> Logical Operator3/5
  Logical Operator9/1 -> Logical Operator3/6
  Logical Operator10/1 -> Logical Operator3/7
  Logical Operator11/1 -> Logical Operator3/8

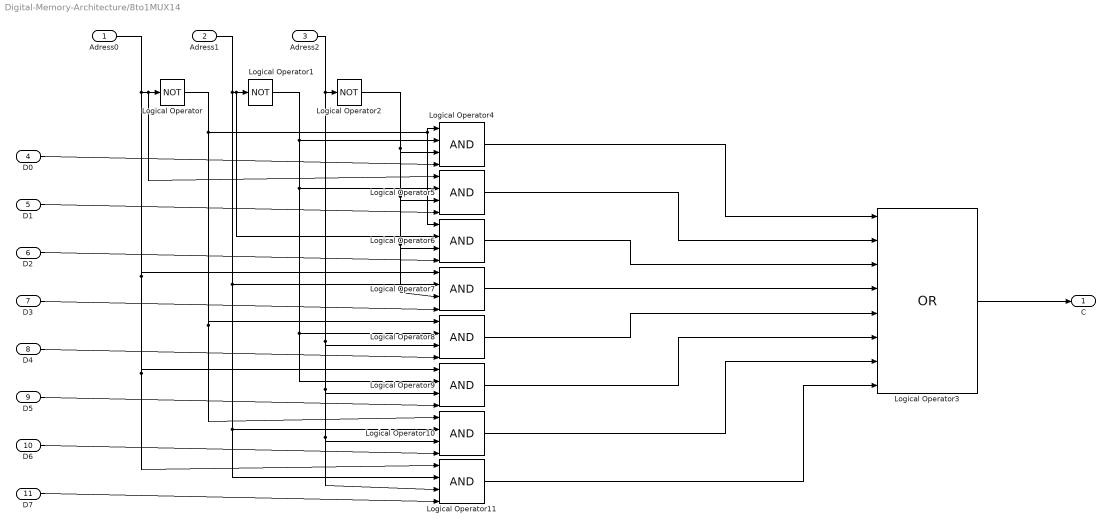
== system Digital-Memory-Architecture/8to1MUX14 ==
  Adress0 : Inport
  Adress1 : Inport  Port=2
  Adress2 : Inport  Port=3
  D0 : Inport  Port=4
  D1 : Inport  Port=5
  D2 : Inport  Port=6
  D3 : Inport  Port=7
  D4 : Inport  Port=8
  D5 : Inport  Port=9
  D6 : Inport  Port=10
  D7 : Inport  Port=11
  Logical Operator : Logic  Operator=NOT  IconShape=distinctive  AllPortsSameDT=off  OutDataTypeStr=boolean
  Logical Operator1 : Logic  Operator=NOT  IconShape=distinctive  AllPortsSameDT=off  OutDataTypeStr=boolean
  Logical Operator{4..11} (8 alike) : Logic  Inputs=4  IconShape=distinctive  AllPortsSameDT=off  OutDataTypeStr=boolean
  Logical Operator2 : Logic  Operator=NOT  IconShape=distinctive  AllPortsSameDT=off  OutDataTypeStr=boolean
  Logical Operator3 : Logic  Operator=OR  Inputs=8  IconShape=distinctive  AllPortsSameDT=off  OutDataTypeStr=boolean
  C : Outport
  wires:
  Logical Operator3/1 -> C/1
  Adress0/1 -> Logical Operator11/1, Logical Operator9/1, Logical Operator7/1, Logical Operator5/1, Logical Operator/1
  Adress1/1 -> Logical Operator11/2, Logical Operator10/2, Logical Operator7/2, Logical Operator6/2, Logical Operator1/1
  Adress2/1 -> Logical Operator11/3, Logical Operator10/3, Logical Operator9/3, Logical Operator8/3, Logical Operator2/1
  D7/1 -> Logical Operator11/4
  D6/1 -> Logical Operator10/4
  D5/1 -> Logical Operator9/4
  D4/1 -> Logical Operator8/4
  D3/1 -> Logical Operator7/4
  D2/1 -> Logical Operator6/4
  D1/1 -> Logical Operator5/4
  D0/1 -> Logical Operator4/4
  Logical Operator2/1 -> Logical Operator7/3, Logical Operator6/3, Logical Operator5/3, Logical Operator4/3
  Logical Operator1/1 -> Logical Operator9/2, Logical Operator8/2, Logical Operator5/2, Logical Operator4/2
  Logical Operator/1 -> Logical Operator10/1, Logical Operator8/1, Logical Operator6/1, Logical Operator4/1
  Logical Operator4/1 -> Logical Operator3/1
  Logical Operator5/1 -> Logical Operator3/2
  Logical Operator6/1 -> Logical Operator3/3
  Logical Operator7/1 -> Logical Operator3/4
  Logical Operator8/1 -> Logical Operator3/5
  Logical Operator9/1 -> Logical Operator3/6
  Logical Operator10/1 -> Logical Operator3/7
  Logical Operator11/1 -> Logical Operator3/8

== system Digital-Memory-Architecture/8to1MUX15 ==
  Adress0 : Inport
  Adress1 : Inport  Port=2
  Adress2 : Inport  Port=3
  D0 : Inport  Port=4
  D1 : Inport  Port=5
  D2 : Inport  Port=6
  D3 : Inport  Port=7
  D4 : Inport  Port=8
  D5 : Inport  Port=9
  D6 : Inport  Port=10
  D7 : Inport  Port=11
  Logical Operator : Logic  Operator=NOT  IconShape=distinctive  AllPortsSameDT=off  OutDataTypeStr=boolean
  Logical Operator1 : Logic  Operator=NOT  IconShape=distinctive  AllPortsSameDT=off  OutDataTypeStr=boolean
  Logical Operator{4..11} (8 alike) : Logic  Inputs=4  IconShape=distinctive  AllPortsSameDT=off  OutDataTypeStr=boolean
  Logical Operator2 : Logic  Operator=NOT  IconShape=distinctive  AllPortsSameDT=off  OutDataTypeStr=boolean
  Logical Operator3 : Logic  Operator=OR  Inputs=8  IconShape=distinctive  AllPortsSameDT=off  OutDataTypeStr=boolean
  D : Outport
  wires:
  Logical Operator3/1 -> D/1
  Adress0/1 -> Logical Operator11/1, Logical Operator9/1, Logical Operator7/1, Logical Operator5/1, Logical Operator/1
  Adress1/1 -> Logical Operator11/2, Logical Operator10/2, Logical Operator7/2, Logical Operator6/2, Logical Operator1/1
  Adress2/1 -> Logical Operator11/3, Logical Operator10/3, Logical Operator9/3, Logical Operator8/3, Logical Operator2/1
  D7/1 -> Logical Operator11/4
  D6/1 -> Logical Operator10/4
  D5/1 -> Logical Operator9/4
  D4/1 -> Logical Operator8/4
  D3/1 -> Logical Operator7/4
  D2/1 -> Logical Operator6/4
  D1/1 -> Logical Operator5/4
  D0/1 -> Logical Operator4/4
  Logical Operator2/1 -> Logical Operator7/3, Logical Operator6/3, Logical Operator5/3, Logical Operator4/3
  Logical Operator1/1 -> Logical Operator9/2, Logical Operator8/2, Logical Operator5/2, Logical Operator4/2
  Logical Operator/1 -> Logical Operator10/1, Logical Operator8/1, Logical Operator6/1, Logical Operator4/1
  Logical Operator4/1 -> Logical Operator3/1
  Logical Operator5/1 -> Logical Operator3/2
  Logical Operator6/1 -> Logical Operator3/3
  Logical Operator7/1 -> Logical Operator3/4
  Logical Operator8/1 -> Logical Operator3/5
  Logical Operator9/1 -> Logical Operator3/6
  Logical Operator10/1 -> Logical Operator3/7
  Logical Operator11/1 -> Logical Operator3/8

== system Digital-Memory-Architecture/8to1MUX2 ==
  Adress0 : Inport
  Adress1 : Inport  Port=2
  Adress2 : Inport  Port=3
  D0 : Inport  Port=4
  D1 : Inport  Port=5
  D2 : Inport  Port=6
  D3 : Inport  Port=7
  D4 : Inport  Port=8
  D5 : Inport  Port=9
  D6 : Inport  Port=10
  D7 : Inport  Port=11
  Logical Operator : Logic  Operator=NOT  IconShape=distinctive  AllPortsSameDT=off  OutDataTypeStr=boolean
  Logical Operator1 : Logic  Operator=NOT  IconShape=distinctive  AllPortsSameDT=off  OutDataTypeStr=boolean
  Logical Operator{4..11} (8 alike) : Logic  Inputs=4  IconShape=distinctive  AllPortsSameDT=off  OutDataTypeStr=boolean
  Logical Operator2 : Logic  Operator=NOT  IconShape=distinctive  AllPortsSameDT=off  OutDataTypeStr=boolean
  Logical Operator3 : Logic  Operator=OR  Inputs=8  IconShape=distinctive  AllPortsSameDT=off  OutDataTypeStr=boolean
  C : Outport
  wires:
  Logical Operator3/1 -> C/1
  Adress0/1 -> Logical Operator11/1, Logical Operator9/1, Logical Operator7/1, Logical Operator5/1, Logical Operator/1
  Adress1/1 -> Logical Operator11/2, Logical Operator10/2, Logical Operator7/2, Logical Operator6/2, Logical Operator1/1
  Adress2/1 -> Logical Operator11/3, Logical Operator10/3, Logical Operator9/3, Logical Operator8/3, Logical Operator2/1
  D7/1 -> Logical Operator11/4
  D6/1 -> Logical Operator10/4
  D5/1 -> Logical Operator9/4
  D4/1 -> Logical Operator8/4
  D3/1 -> Logical Operator7/4
  D2/1 -> Logical Operator6/4
  D1/1 -> Logical Operator5/4
  D0/1 -> Logical Operator4/4
  Logical Operator2/1 -> Logical Operator7/3, Logical Operator6/3, Logical Operator5/3, Logical Operator4/3
  Logical Operator1/1 -> Logical Operator9/2, Logical Operator8/2, Logical Operator5/2, Logical Operator4/2
  Logical Operator/1 -> Logical Operator10/1, Logical Operator8/1, Logical Operator6/1, Logical Operator4/1
  Logical Operator4/1 -> Logical Operator3/1
  Logical Operator5/1 -> Logical Operator3/2
  Logical Operator6/1 -> Logical Operator3/3
  Logical Operator7/1 -> Logical Operator3/4
  Logical Operator8/1 -> Logical Operator3/5
  Logical Operator9/1 -> Logical Operator3/6
  Logical Operator10/1 -> Logical Operator3/7
  Logical Operator11/1 -> Logical Operator3/8

== system Digital-Memory-Architecture/8to1MUX3 ==
  Adress0 : Inport
  Adress1 : Inport  Port=2
  Adress2 : Inport  Port=3
  D0 : Inport  Port=4
  D1 : Inport  Port=5
  D2 : Inport  Port=6
  D3 : Inport  Port=7
  D4 : Inport  Port=8
  D5 : Inport  Port=9
  D6 : Inport  Port=10
  D7 : Inport  Port=11
  Logical Operator : Logic  Operator=NOT  IconShape=distinctive  AllPortsSameDT=off  OutDataTypeStr=boolean
  Logical Operator1 : Logic  Operator=NOT  IconShape=distinctive  AllPortsSameDT=off  OutDataTypeStr=boolean
  Logical Operator{4..11} (8 alike) : Logic  Inputs=4  IconShape=distinctive  AllPortsSameDT=off  OutDataTypeStr=boolean
  Logical Operator2 : Logic  Operator=NOT  IconShape=distinctive  AllPortsSameDT=off  OutDataTypeStr=boolean
  Logical Operator3 : Logic  Operator=OR  Inputs=8  IconShape=distinctive  AllPortsSameDT=off  OutDataTypeStr=boolean
  D : Outport
  wires:
  Logical Operator3/1 -> D/1
  Adress0/1 -> Logical Operator11/1, Logical Operator9/1, Logical Operator7/1, Logical Operator5/1, Logical Operator/1
  Adress1/1 -> Logical Operator11/2, Logical Operator10/2, Logical Operator7/2, Logical Operator6/2, Logical Operator1/1
  Adress2/1 -> Logical Operator11/3, Logical Operator10/3, Logical Operator9/3, Logical Operator8/3, Logical Operator2/1
  D7/1 -> Logical Operator11/4
  D6/1 -> Logical Operator10/4
  D5/1 -> Logical Operator9/4
  D4/1 -> Logical Operator8/4
  D3/1 -> Logical Operator7/4
  D2/1 -> Logical Operator6/4
  D1/1 -> Logical Operator5/4
  D0/1 -> Logical Operator4/4
  Logical Operator2/1 -> Logical Operator7/3, Logical Operator6/3, Logical Operator5/3, Logical Operator4/3
  Logical Operator1/1 -> Logical Operator9/2, Logical Operator8/2, Logical Operator5/2, Logical Operator4/2
  Logical Operator/1 -> Logical Operator10/1, Logical Operator8/1, Logical Operator6/1, Logical Operator4/1
  Logical Operator4/1 -> Logical Operator3/1
  Logical Operator5/1 -> Logical Operator3/2
  Logical Operator6/1 -> Logical Operator3/3
  Logical Operator7/1 -> Logical Operator3/4
  Logical Operator8/1 -> Logical Operator3/5
  Logical Operator9/1 -> Logical Operator3/6
  Logical Operator10/1 -> Logical Operator3/7
  Logical Operator11/1 -> Logical Operator3/8

== system Digital-Memory-Architecture/8to1MUX4 ==
  Adress0 : Inport
  Adress1 : Inport  Port=2
  Adress2 : Inport  Port=3
  D0 : Inport  Port=4
  D1 : Inport  Port=5
  D2 : Inport  Port=6
  D3 : Inport  Port=7
  D4 : Inport  Port=8
  D5 : Inport  Port=9
  D6 : Inport  Port=10
  D7 : Inport  Port=11
  Logical Operator : Logic  Operator=NOT  IconShape=distinctive  AllPortsSameDT=off  OutDataTypeStr=boolean
  Logical Operator1 : Logic  Operator=NOT  IconShape=distinctive  AllPortsSameDT=off  OutDataTypeStr=boolean
  Logical Operator{4..11} (8 alike) : Logic  Inputs=4  IconShape=distinctive  AllPortsSameDT=off  OutDataTypeStr=boolean
  Logical Operator2 : Logic  Operator=NOT  IconShape=distinctive  AllPortsSameDT=off  OutDataTypeStr=boolean
  Logical Operator3 : Logic  Operator=OR  Inputs=8  IconShape=distinctive  AllPortsSameDT=off  OutDataTypeStr=boolean
  A : Outport
  wires:
  Logical Operator3/1 -> A/1
  Adress0/1 -> Logical Operator11/1, Logical Operator9/1, Logical Operator7/1, Logical Operator5/1, Logical Operator/1
  Adress1/1 -> Logical Operator11/2, Logical Operator10/2, Logical Operator7/2, Logical Operator6/2, Logical Operator1/1
  Adress2/1 -> Logical Operator11/3, Logical Operator10/3, Logical Operator9/3, Logical Operator8/3, Logical Operator2/1
  D7/1 -> Logical Operator11/4
  D6/1 -> Logical Operator10/4
  D5/1 -> Logical Operator9/4
  D4/1 -> Logical Operator8/4
  D3/1 -> Logical Operator7/4
  D2/1 -> Logical Operator6/4
  D1/1 -> Logical Operator5/4
  D0/1 -> Logical Operator4/4
  Logical Operator2/1 -> Logical Operator7/3, Logical Operator6/3, Logical Operator5/3, Logical Operator4/3
  Logical Operator1/1 -> Logical Operator9/2, Logical Operator8/2, Logical Operator5/2, Logical Operator4/2
  Logical Operator/1 -> Logical Operator10/1, Logical Operator8/1, Logical Operator6/1, Logical Operator4/1
  Logical Operator4/1 -> Logical Operator3/1
  Logical Operator5/1 -> Logical Operator3/2
  Logical Operator6/1 -> Logical Operator3/3
  Logical Operator7/1 -> Logical Operator3/4
  Logical Operator8/1 -> Logical Operator3/5
  Logical Operator9/1 -> Logical Operator3/6
  Logical Operator10/1 -> Logical Operator3/7
  Logical Operator11/1 -> Logical Operator3/8

== system Digital-Memory-Architecture/8to1MUX5 ==
  Adress0 : Inport
  Adress1 : Inport  Port=2
  Adress2 : Inport  Port=3
  D0 : Inport  Port=4
  D1 : Inport  Port=5
  D2 : Inport  Port=6
  D3 : Inport  Port=7
  D4 : Inport  Port=8
  D5 : Inport  Port=9
  D6 : Inport  Port=10
  D7 : Inport  Port=11
  Logical Operator : Logic  Operator=NOT  IconShape=distinctive  AllPortsSameDT=off  OutDataTypeStr=boolean
  Logical Operator1 : Logic  Operator=NOT  IconShape=distinctive  AllPortsSameDT=off  OutDataTypeStr=boolean
  Logical Operator{4..11} (8 alike) : Logic  Inputs=4  IconShape=distinctive  AllPortsSameDT=off  OutDataTypeStr=boolean
  Logical Operator2 : Logic  Operator=NOT  IconShape=distinctive  AllPortsSameDT=off  OutDataTypeStr=boolean
  Logical Operator3 : Logic  Operator=OR  Inputs=8  IconShape=distinctive  AllPortsSameDT=off  OutDataTypeStr=boolean
  B : Outport
  wires:
  Logical Operator3/1 -> B/1
  Adress0/1 -> Logical Operator11/1, Logical Operator9/1, Logical Operator7/1, Logical Operator5/1, Logical Operator/1
  Adress1/1 -> Logical Operator11/2, Logical Operator10/2, Logical Operator7/2, Logical Operator6/2, Logical Operator1/1
  Adress2/1 -> Logical Operator11/3, Logical Operator10/3, Logical Operator9/3, Logical Operator8/3, Logical Operator2/1
  D7/1 -> Logical Operator11/4
  D6/1 -> Logical Operator10/4
  D5/1 -> Logical Operator9/4
  D4/1 -> Logical Operator8/4
  D3/1 -> Logical Operator7/4
  D2/1 -> Logical Operator6/4
  D1/1 -> Logical Operator5/4
  D0/1 -> Logical Operator4/4
  Logical Operator2/1 -> Logical Operator7/3, Logical Operator6/3, Logical Operator5/3, Logical Operator4/3
  Logical Operator1/1 -> Logical Operator9/2, Logical Operator8/2, Logical Operator5/2, Logical Operator4/2
  Logical Operator/1 -> Logical Operator10/1, Logical Operator8/1, Logical Operator6/1, Logical Operator4/1
  Logical Operator4/1 -> Logical Operator3/1
  Logical Operator5/1 -> Logical Operator3/2
  Logical Operator6/1 -> Logical Operator3/3
  Logical Operator7/1 -> Logical Operator3/4
  Logical Operator8/1 -> Logical Operator3/5
  Logical Operator9/1 -> Logical Operator3/6
  Logical Operator10/1 -> Logical Operator3/7
  Logical Operator11/1 -> Logical Operator3/8

== system Digital-Memory-Architecture/8to1MUX6 ==
  Adress0 : Inport
  Adress1 : Inport  Port=2
  Adress2 : Inport  Port=3
  D0 : Inport  Port=4
  D1 : Inport  Port=5
  D2 : Inport  Port=6
  D3 : Inport  Port=7
  D4 : Inport  Port=8
  D5 : Inport  Port=9
  D6 : Inport  Port=10
  D7 : Inport  Port=11
  Logical Operator : Logic  Operator=NOT  IconShape=distinctive  AllPortsSameDT=off  OutDataTypeStr=boolean
  Logical Operator1 : Logic  Operator=NOT  IconShape=distinctive  AllPortsSameDT=off  OutDataTypeStr=boolean
  Logical Operator{4..11} (8 alike) : Logic  Inputs=4  IconShape=distinctive  AllPortsSameDT=off  OutDataTypeStr=boolean
  Logical Operator2 : Logic  Operator=NOT  IconShape=distinctive  AllPortsSameDT=off  OutDataTypeStr=boolean
  Logical Operator3 : Logic  Operator=OR  Inputs=8  IconShape=distinctive  AllPortsSameDT=off  OutDataTypeStr=boolean
  C : Outport
  wires:
  Logical Operator3/1 -> C/1
  Adress0/1 -> Logical Operator11/1, Logical Operator9/1, Logical Operator7/1, Logical Operator5/1, Logical Operator/1
  Adress1/1 -> Logical Operator11/2, Logical Operator10/2, Logical Operator7/2, Logical Operator6/2, Logical Operator1/1
  Adress2/1 -> Logical Operator11/3, Logical Operator10/3, Logical Operator9/3, Logical Operator8/3, Logical Operator2/1
  D7/1 -> Logical Operator11/4
  D6/1 -> Logical Operator10/4
  D5/1 -> Logical Operator9/4
  D4/1 -> Logical Operator8/4
  D3/1 -> Logical Operator7/4
  D2/1 -> Logical Operator6/4
  D1/1 -> Logical Operator5/4
  D0/1 -> Logical Operator4/4
  Logical Operator2/1 -> Logical Operator7/3, Logical Operator6/3, Logical Operator5/3, Logical Operator4/3
  Logical Operator1/1 -> Logical Operator9/2, Logical Operator8/2, Logical Operator5/2, Logical Operator4/2
  Logical Operator/1 -> Logical Operator10/1, Logical Operator8/1, Logical Operator6/1, Logical Operator4/1
  Logical Operator4/1 -> Logical Operator3/1
  Logical Operator5/1 -> Logical Operator3/2
  Logical Operator6/1 -> Logical Operator3/3
  Logical Operator7/1 -> Logical Operator3/4
  Logical Operator8/1 -> Logical Operator3/5
  Logical Operator9/1 -> Logical Operator3/6
  Logical Operator10/1 -> Logical Operator3/7
  Logical Operator11/1 -> Logical Operator3/8
